simulink model "waypoint_generation_ptCloud_200726_mapdata_filtering_4m_2"  (R2020a)
settings: Solver=ode4  StartTime=0.0  StopTime=150  FixedStep=0.01  RelTol=1e-3  EnableMultiTasking=on
InitFcn:
  | detector = load('ptOPDetector.mat');
  | OPdetector = detector.OPdetector;
undefined symbols (not defined in the file): g, Kd_p, Kd_q, Kd_r, Kd_vx, Kd_vy, Kd_vz, Kff_r, Kff_vx, Kff_vy, Kff_vz, Ki_p, Ki_q, Ki_r, Ki_vx, Ki_vy, Ki_vz, Kp_p, Kp_phi, Kp_psi, Kp_q, Kp_r, Kp_theta, Kp_vx, Kp_vy, Kp_vz, M, pointCloud_center, sigma_motor, w_h
libraries: visiontextngfix x4, sharedtransform x1, shared6dof x1, simulink_extras x1
(part 1 of 3)
settings Model: Creator=WIN7  LastModifiedBy=USER
settings DataIOCC: LimitDataPoints=on  ReturnWorkspaceOutputs=off
settings OptimizationCC: LifeSpan=inf
settings DebuggingCC: AllowSymbolicDim=off  SFUnexpectedBacktrackingDiag=warning  SFNoUnconditionalDefaultTransitionDiag=warning  SFExecutionAtInitializationDiag=none  ArithmeticOperatorsInVariantConditions=warning
settings ModelReferenceCC: PropagateSignalLabelsOutOfModel=off
settings SFSimCC: SimUseLocalCustomCode=off  CustomCodeUndefinedFunction=UseInterfaceOnly
settings RTWCC: RTWUseLocalCustomCode=off
settings CodeAppCC: StateflowObjectComments=on
settings GRTTargetCC: TargetLangStandard=C89/C90 (ANSI)
settings ConfigComp: CovMetricSettings=dw  CovHtmlReporting=on  CovSaveCumulativeToWorkspaceVar=on  CovSaveSingleToWorkspaceVar=on  CovExternalEMLEnable=off

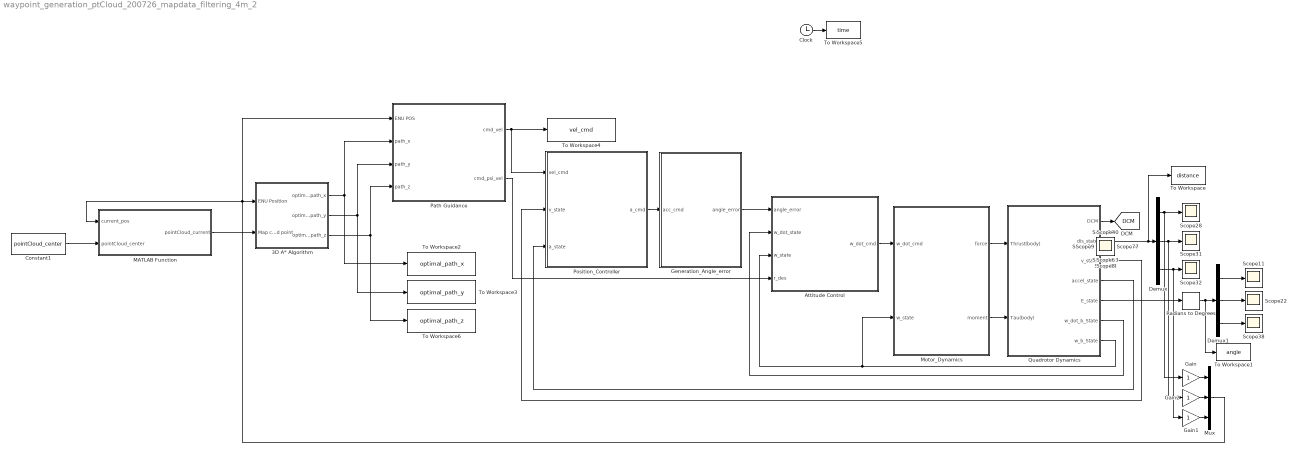
== system waypoint_generation_ptCloud_200726_mapdata_filtering_4m_2 ==
  3D A* Algorithm : Subsystem
  Attitude Control : Subsystem
  Clock : Clock
  Constant1 : Constant  Value=pointCloud_center
  Demux : Demux  Outputs=3
  Demux1 : Demux  Outputs=3
  Gain : Gain
  Gain1 : Gain
  Gain2 : Gain
  Generation_Angle_error : Subsystem
  MATLAB Function : MATLAB Function  TreatAsAtomicUnit=on
  Motor_Dynamics : Subsystem
  Mux : Mux  Inputs=3
  Path Guidance : Subsystem
  Position_Controller : Subsystem
  Quadrotor Dynamics : Subsystem
  Radians to Degrees : simulink_extras/Transformations/Radians to Degrees
  Scope{,1..40} (41 alike) : Scope
  To Workspace : ToWorkspace  VariableName=distance  SampleTime=-1
  To Workspace1 : ToWorkspace  VariableName=angle  SampleTime=-1
  To Workspace2 : ToWorkspace  VariableName=optimal_path_x  SampleTime=-1
  To Workspace3 : ToWorkspace  VariableName=optimal_path_y  SampleTime=-1
  To Workspace4 : ToWorkspace  VariableName=vel_cmd  SampleTime=-1
  To Workspace5 : ToWorkspace  VariableName=time  SampleTime=-1
  To Workspace6 : ToWorkspace  VariableName=optimal_path_z  SampleTime=-1
  tag scope: DCM=global
  wires:
  Quadrotor Dynamics/7(w_b_State) -> Attitude Control/3(w_state), Motor_Dynamics/2(w_state)
  Quadrotor Dynamics/6(w_dot_b_State) -> Attitude Control/2(w_dot_state)
  Quadrotor Dynamics/1(DCM) -> [DCM]
  Demux/1 -> Scope28/1, Gain/1
  Demux/3 -> Scope32/1, Gain1/1
  Demux/2 -> Scope31/1, Gain2/1
  Generation_Angle_error/1(angle_error) -> Attitude Control/1(angle_error)
  Position_Controller/1(a_cmd) -> Generation_Angle_error/1(acc_cmd)
  Quadrotor Dynamics/3(v_state) -> Position_Controller/2(v_state)
  Quadrotor Dynamics/4(accel_state) -> Position_Controller/3(a_state)
  Attitude Control/1(w_dot_cmd) -> Motor_Dynamics/1(w_dot_cmd)
  Motor_Dynamics/1(force) -> Quadrotor Dynamics/1(Thrust(body))
  Motor_Dynamics/2(moment) -> Quadrotor Dynamics/2(Tau(body))
  Demux1/1 -> Scope11/1
  Demux1/3 -> Scope38/1
  Demux1/2 -> Scope22/1
  Quadrotor Dynamics/5(E_state) -> Radians to Degrees/1
  Clock/1 -> To Workspace5/1
  Radians to Degrees/1 -> To Workspace1/1, Demux1/1
  Quadrotor Dynamics/2(dis_state) -> To Workspace/1, Demux/1
  Path Guidance/1(cmd_vel) -> Position_Controller/1("vel_cmd "), To Workspace4/1
  3D A* Algorithm/1(optimal_path_x) -> Path Guidance/2(path_x), To Workspace2/1
  3D A* Algorithm/2(optimal_path_y) -> Path Guidance/3(path_y), To Workspace3/1
  3D A* Algorithm/3(optimal_path_z) -> Path Guidance/4(path_z), To Workspace6/1
  Gain2/1 -> Mux/2
  Gain1/1 -> Mux/3
  Mux/1 -> Path Guidance/1("ENU POS "), MATLAB Function/1(current_pos), 3D A* Algorithm/1(ENU Position)
  Path Guidance/2("cmd_psi_vel ") -> Attitude Control/4("r_des ")
  Gain/1 -> Mux/1
  Constant1/1 -> MATLAB Function/2(pointCloud_center)
  MATLAB Function/1(pointCloud_current) -> 3D A* Algorithm/2(Map cloud point)

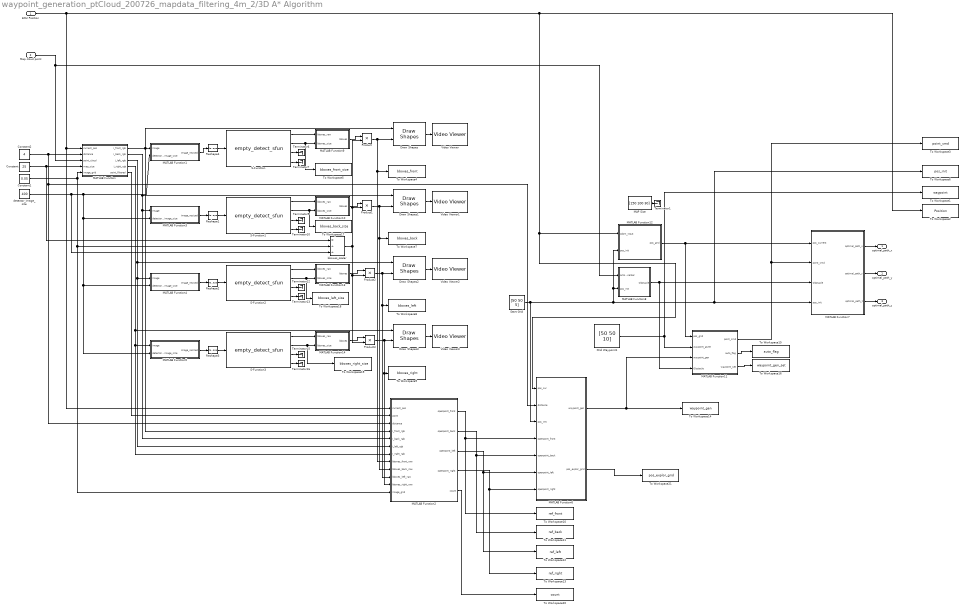
== system waypoint_generation_ptCloud_200726_mapdata_filtering_4m_2/3D A* Algorithm ==
  ENU Position : Inport
  Map cloud point : Inport  Port=2
  Constant : Constant  Value=25
  Constant1 : Constant  Value=0.05
  Constant2 : Constant  Value=4
  Draw Shapes{,1..3} (4 alike) : visiontextngfix/Draw Shapes  shape=Rectangles  fill=off  lineWidth=4  fillClrSource=Specify via dialog  display=User-specified value  intensity=200  color=[255 255 0]  opacity=0.6  viewport=Entire image  antialiasing=off  inType=Obsolete  imagePorts=One multidimensional signal  roundingMode=Floor  overflowMode=off  memoryMode=Specify word length  memoryWordLength=16  prodOutputMode=Binary point scaling  prodOutputWordLength=32  prodOutputFracLength=14  memoryFracLength=14
  Grid Waypoint1 : Constant  Value=[50 50 10]  VectorParams1D=off
  MAP Size : Constant  Value=[150 100 30]
  MATLAB Function : MATLAB Function  TreatAsAtomicUnit=on
  MATLAB Function1 : MATLAB Function  TreatAsAtomicUnit=on
  MATLAB Function10 : MATLAB Function  TreatAsAtomicUnit=on
  MATLAB Function11 : MATLAB Function  TreatAsAtomicUnit=on
  MATLAB Function12 : MATLAB Function  TreatAsAtomicUnit=on
  MATLAB Function13 : MATLAB Function  TreatAsAtomicUnit=on
  MATLAB Function14 : MATLAB Function  TreatAsAtomicUnit=on
  MATLAB Function2 : MATLAB Function  TreatAsAtomicUnit=on
  MATLAB Function3 : MATLAB Function  TreatAsAtomicUnit=on
  MATLAB Function4 : MATLAB Function  TreatAsAtomicUnit=on
  MATLAB Function5 : MATLAB Function  TreatAsAtomicUnit=on
  MATLAB Function6 : MATLAB Function  TreatAsAtomicUnit=on
  MATLAB Function7 : MATLAB Function  TreatAsAtomicUnit=on
  MATLAB Function8 : MATLAB Function  TreatAsAtomicUnit=on
  MATLAB Function9 : MATLAB Function  TreatAsAtomicUnit=on
  Product{,1..3} (4 alike) : Product
  Reshape{1..4} (4 alike) : Reshape
  S-Function{,1..3} (4 alike) : S-Function  FunctionName=empty_detect_sfun  SFunctionDeploymentMode=off  EnableBusSupport=off
  Start Grid : Constant  Value=[50 50 5]
  Terminator{1,6..7,9..10,12..13,15..16} (9 alike) : Terminator
  To Workspace1 : ToWorkspace  VariableName=waypoint  SampleTime=-1
      settings: Save2DSignal=2-D array (concatenate along first dimension)
  To Workspace10 : ToWorkspace  VariableName=ref_front  SampleTime=-1
  To Workspace11 : ToWorkspace  VariableName=ref_back  SampleTime=-1
  To Workspace12 : ToWorkspace  VariableName=ref_left  SampleTime=-1
  To Workspace13 : ToWorkspace  VariableName=ref_right  SampleTime=-1
  To Workspace14 : ToWorkspace  VariableName=waypoint_gen  SampleTime=-1
  To Workspace15 : ToWorkspace  VariableName=auto_flag  SampleTime=-1
  To Workspace16 : ToWorkspace  VariableName=waypoint_gen_set  SampleTime=-1
  To Workspace17 : ToWorkspace  VariableName=bboxes_back_size  SampleTime=-1
  To Workspace18 : ToWorkspace  VariableName=bboxes_left_size  SampleTime=-1
  To Workspace19 : ToWorkspace  VariableName=bboxes_right_size  SampleTime=-1
  To Workspace2 : ToWorkspace  VariableName=Position  SampleTime=-1
  To Workspace20 : ToWorkspace  VariableName=count  SampleTime=-1
  To Workspace21 : ToWorkspace  VariableName=pos_explor_grid  SampleTime=-1
  To Workspace3 : ToWorkspace  VariableName=point_cmd  SampleTime=-1
      settings: Save2DSignal=2-D array (concatenate along first dimension)
  To Workspace4 : ToWorkspace  VariableName=bboxes_front  SampleTime=-1
  To Workspace5 : ToWorkspace  VariableName=bboxes_front_size  SampleTime=-1
  To Workspace6 : ToWorkspace  VariableName=pos_init  SampleTime=-1
      settings: Save2DSignal=2-D array (concatenate along first dimension)
  To Workspace7 : ToWorkspace  VariableName=bboxes_back  SampleTime=-1
  To Workspace8 : ToWorkspace  VariableName=bboxes_left  SampleTime=-1
  To Workspace9 : ToWorkspace  VariableName=bboxes_right  SampleTime=-1
  Video Viewer : VideoViewer  FigPos=[7 678 732 569]
  Video Viewer1 : VideoViewer  FigPos=[742 680 732 569]
  Video Viewer2 : VideoViewer  FigPos=[0 1098 732 569]
  Video Viewer3 : VideoViewer  FigPos=[646 1041 732 569]
  bboxes_scalar : Product  Inputs=*//
  detector_image_size : Constant  Value=400
  optimal_path_x : Outport  VectorParamsAs1DForOutWhenUnconnected=off
  optimal_path_y : Outport  Port=2  VectorParamsAs1DForOutWhenUnconnected=off
  optimal_path_z : Outport  Port=3  VectorParamsAs1DForOutWhenUnconnected=off
  wires:
  MATLAB Function8/1(Obstacle) -> MATLAB Function11/4(Obstacle), MATLAB Function7/3(Obstacle)
  MATLAB Function12/1(pos_grid) -> MATLAB Function7/1(pos_current), MATLAB Function11/1(pos_grid)
  Start Grid/1 -> To Workspace6/1, MATLAB Function7/4(pos_init), MATLAB Function12/2(pos_init), MATLAB Function8/2(pos_init), MATLAB Function6/3(pos_init)
  MATLAB Function11/1(point_cmd) -> MATLAB Function7/2(point_cmd), To Workspace3/1
  MAP Size/1 -> Terminator1/1
  MATLAB Function7/1(optimal_path_x) -> optimal_path_x/1
  MATLAB Function7/2(optimal_path_y) -> optimal_path_y/1
  MATLAB Function7/3(optimal_path_z) -> optimal_path_z/1
  ENU Position/1 -> To Workspace2/1, MATLAB Function6/1(pos_cur), MATLAB Function12/1(odom_input), MATLAB Function2/1(current_pos), MATLAB Function/1(current_pos)
  Map cloud point/1 -> MATLAB Function8/1(octomap_center), MATLAB Function/3(point_cloud)
  Grid Waypoint1/1 -> To Workspace1/1, MATLAB Function11/2(waypoint_given)
  MATLAB Function/2(I_back_rgb) -> MATLAB Function2/5(I_back_rgb), MATLAB Function3/1(Image), Draw Shapes1/1
  MATLAB Function/3(I_left_rgb) -> MATLAB Function2/6(I_left_rgb), MATLAB Function4/1(Image), Draw Shapes2/1
  MATLAB Function1/1(Image_resized) -> Reshape4/1
  S-Function/2 -> To Workspace5/1, MATLAB Function9/2(bboxes_size)
  S-Function/4 -> Terminator7/1
  S-Function/3 -> Terminator6/1
  Reshape4/1 -> S-Function/1
  S-Function/1 -> MATLAB Function9/1(bboxes_raw)
  MATLAB Function/4(I_right_rgb) -> MATLAB Function2/7(I_right_rgb), MATLAB Function5/1(Image), Draw Shapes3/1
  S-Function1/3 -> Terminator9/1
  S-Function1/2 -> To Workspace17/1, MATLAB Function10/2(bboxes_size)
  MATLAB Function3/1(Image_resized) -> Reshape1/1
  S-Function1/4 -> Terminator10/1
  Reshape1/1 -> S-Function1/1
  S-Function1/1 -> MATLAB Function10/1(bboxes_raw)
  S-Function2/3 -> Terminator12/1
  S-Function2/2 -> To Workspace18/1, MATLAB Function13/2(bboxes_size)
  MATLAB Function4/1(Image_resized) -> Reshape2/1
  S-Function2/4 -> Terminator13/1
  Reshape2/1 -> S-Function2/1
  S-Function2/1 -> MATLAB Function13/1(bboxes_raw)
  S-Function3/3 -> Terminator15/1
  MATLAB Function5/1(Image_resized) -> Reshape3/1
  S-Function3/4 -> Terminator16/1
  Reshape3/1 -> S-Function3/1
  MATLAB Function2/4(openpoint_right) -> MATLAB Function6/7(openpoint_right), To Workspace13/1
  MATLAB Function2/3(openpoint_left) -> MATLAB Function6/6(openpoint_left), To Workspace12/1
  MATLAB Function2/1(openpoint_front) -> MATLAB Function6/4(openpoint_front), To Workspace10/1
  MATLAB Function2/2(openpoint_back) -> MATLAB Function6/5(openpoint_back), To Workspace11/1
  Draw Shapes/1 -> Video Viewer/1
  MATLAB Function/1(I_front_rgb) -> MATLAB Function2/4(I_front_rgb), Draw Shapes/1, MATLAB Function1/1(Image)
  Product/1 -> Draw Shapes/2, MATLAB Function2/8(bboxes_front_raw), To Workspace4/1
  Product1/1 -> MATLAB Function2/9(bboxes_back_raw), To Workspace7/1, Draw Shapes1/2
  Draw Shapes1/1 -> Video Viewer1/1
  Product2/1 -> Draw Shapes2/2, MATLAB Function2/10(bboxes_left_raw), To Workspace8/1
  Draw Shapes2/1 -> Video Viewer2/1
  Product3/1 -> Draw Shapes3/2, MATLAB Function2/11(bboxes_right_raw), To Workspace9/1
  Draw Shapes3/1 -> Video Viewer3/1
  MATLAB Function6/1(waypoint_gen) -> MATLAB Function11/3(waypoint_gen), To Workspace14/1
  MATLAB Function11/2(auto_flag) -> To Workspace15/1
  MATLAB Function11/3(waypoint_set) -> To Workspace16/1
  S-Function3/2 -> To Workspace19/1, MATLAB Function14/2(bboxes_size)
  S-Function3/1 -> MATLAB Function14/1(bboxes_raw)
  Constant/1 -> bboxes_scalar/1, MATLAB Function/4(map_size)
  Constant1/1 -> MATLAB Function2/12(image_grid), bboxes_scalar/2, MATLAB Function/5(image_grid)
  detector_image_size/1 -> bboxes_scalar/3, MATLAB Function5/2(detector_image_size), MATLAB Function4/2(detector_image_size), MATLAB Function3/2(detector_image_size), MATLAB Function1/2(detector_image_size)
  MATLAB Function9/1(bboxes) -> Product/1
  bboxes_scalar/1 -> Product3/2, Product2/2, Product1/2, Product/2
  MATLAB Function10/1(bboxes) -> Product1/1
  MATLAB Function13/1(bboxes) -> Product2/1
  MATLAB Function14/1(bboxes) -> Product3/1
  MATLAB Function2/5(count) -> To Workspace20/1
  MATLAB Function6/2(pos_explor_grid) -> To Workspace21/1
  Constant2/1 -> MATLAB Function6/2(distance), MATLAB Function2/3(distance), MATLAB Function/2(distance)
  MATLAB Function/5(point_filtered) -> MATLAB Function2/2(point)

== system waypoint_generation_ptCloud_200726_mapdata_filtering_4m_2/Attitude Control ==
  angle_error : Inport
  w_dot_state : Inport  Port=2
  w_state : Inport  Port=3
  "r_des " : Inport  Port=4
  Angle controller : Subsystem
  Angular velocity controller : Subsystem
  Mux1 : Mux  Inputs=3
  Step3 : Step  Time=0  After=0  SampleTime=0
  Step4 : Step  Time=0  After=0.002  SampleTime=0
  Step5 : Step  Time=0  After=0.005  SampleTime=0
  w_dot_cmd : Outport  VectorParamsAs1DForOutWhenUnconnected=off
  wires:
  angle_error/1 -> Angle controller/1(E_des)
  w_dot_state/1 -> Angular velocity controller/3(w_dot_state)
  w_state/1 -> Angular velocity controller/2(w_state)
  Step3/1 -> Mux1/1
  Step4/1 -> Mux1/2
  Step5/1 -> Mux1/3
  Angular velocity controller/1(w_dot_cmd) -> w_dot_cmd/1
  Angle controller/1(w_cmd) -> Angular velocity controller/1(w_cmd)
  "r_des "/1 -> Angular velocity controller/4("r_des ")

== system waypoint_generation_ptCloud_200726_mapdata_filtering_4m_2/Generation_Angle_error ==
  acc_cmd : Inport
  Attitude Generation (phi,theta,psi) : MATLAB Function  TreatAsAtomicUnit=on
  Attitude Generation(phi,theta,psi^*) : MATLAB Function  TreatAsAtomicUnit=on
  Attitude Generation(psi^*) : MATLAB Function  TreatAsAtomicUnit=on
  Constant : Constant  Value=0
  angle_error : Outport  VectorParamsAs1DForOutWhenUnconnected=off
  wires:
  [DCM] -> Attitude Generation (phi,theta,psi)/1(DCM)
  Attitude Generation (phi,theta,psi)/2(R_rp_x) -> Attitude Generation(psi^*)/1(R_rp_x)
  acc_cmd/1 -> Attitude Generation(psi^*)/2(acc_cmd), Attitude Generation (phi,theta,psi)/2(acc_cmd)
  Attitude Generation(phi,theta,psi^*)/1(angle_error_result) -> angle_error/1
  Attitude Generation (phi,theta,psi)/1(angle_error) -> Attitude Generation(phi,theta,psi^*)/1(angle_error)
  Attitude Generation(psi^*)/1(psi_angle_error) -> Attitude Generation(phi,theta,psi^*)/2(psi_angle_error)
  Constant/1 -> Attitude Generation(psi^*)/3(Bearing_angle)

== system waypoint_generation_ptCloud_200726_mapdata_filtering_4m_2/Motor_Dynamics ==
  w_dot_cmd : Inport
  w_state : Inport  Port=2
  Motor Dynamics : Subsystem
  "Thrust &  Moment Generation " : MATLAB Function  TreatAsAtomicUnit=on
  force : Outport  VectorParamsAs1DForOutWhenUnconnected=off
  moment : Outport  Port=2  VectorParamsAs1DForOutWhenUnconnected=off
  wires:
  "Thrust &  Moment Generation "/2(moment) -> moment/1
  "Thrust &  Moment Generation "/1(force) -> force/1
  Motor Dynamics/1(w_com) -> "Thrust &  Moment Generation "/1(w_des_nomal)
  w_dot_cmd/1 -> Motor Dynamics/1(w_dot_cmd)
  w_state/1 -> Motor Dynamics/2(w_state)

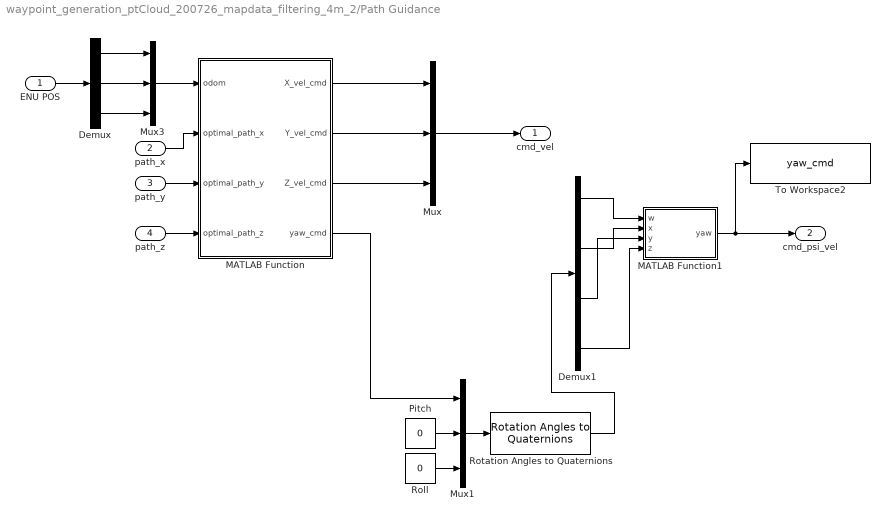
== system waypoint_generation_ptCloud_200726_mapdata_filtering_4m_2/Path Guidance ==
  "ENU POS " : Inport
  path_x : Inport  Port=2
  path_y : Inport  Port=3
  path_z : Inport  Port=4
  " Roll" : Constant  Value=0  OutDataTypeStr=double  SampleTime=-1
  Demux : Demux  Outputs=3
  Demux1 : Demux
  MATLAB Function : MATLAB Function  TreatAsAtomicUnit=on
  MATLAB Function1 : MATLAB Function  TreatAsAtomicUnit=on
  Mux : Mux  Inputs=3
  Mux1 : Mux  Inputs=3
  Mux3 : Mux  Inputs=3
  Pitch : Constant  Value=0  OutDataTypeStr=double  SampleTime=-1
  Rotation Angles to Quaternions : sharedtransform/Rotation Angles to Quaternions  rotationOrder=ZYX  aMode=aMode
      settings: SourceProductBaseCode=AE,PW,MT,VE,VP
  To Workspace2 : ToWorkspace  VariableName=yaw_cmd  SampleTime=-1
  cmd_vel : Outport  VectorParamsAs1DForOutWhenUnconnected=off
  "cmd_psi_vel " : Outport  Port=2  VectorParamsAs1DForOutWhenUnconnected=off
  wires:
  MATLAB Function/3(Z_vel_cmd) -> Mux/3
  path_y/1 -> MATLAB Function/3(optimal_path_y)
  Mux3/1 -> MATLAB Function/1(odom)
  path_z/1 -> MATLAB Function/4(optimal_path_z)
  path_x/1 -> MATLAB Function/2(optimal_path_x)
  Mux/1 -> cmd_vel/1
  "ENU POS "/1 -> Demux/1
  Demux/1 -> Mux3/1
  Demux/2 -> Mux3/2
  Demux/3 -> Mux3/3
  MATLAB Function/1(X_vel_cmd) -> Mux/1
  MATLAB Function/2(Y_vel_cmd) -> Mux/2
  Demux1/4 -> MATLAB Function1/4(z)
  " Roll"/1 -> Mux1/3
  Mux1/1 -> Rotation Angles to Quaternions/1
  MATLAB Function/4(yaw_cmd) -> Mux1/1
  Pitch/1 -> Mux1/2
  Rotation Angles to Quaternions/1 -> Demux1/1
  Demux1/3 -> MATLAB Function1/3(y)
  Demux1/1 -> MATLAB Function1/1(w)
  Demux1/2 -> MATLAB Function1/2(x)
  MATLAB Function1/1(yaw) -> To Workspace2/1, "cmd_psi_vel "/1

== system waypoint_generation_ptCloud_200726_mapdata_filtering_4m_2/Position_Controller ==
  "vel_cmd " : Inport
  v_state : Inport  Port=2
  a_state : Inport  Port=3
  Velocity Controller : Subsystem
  a_cmd : Outport  VectorParamsAs1DForOutWhenUnconnected=off
  wires:
  Velocity Controller/1(a_cmd) -> a_cmd/1
  v_state/1 -> Velocity Controller/2(v_state)
  a_state/1 -> Velocity Controller/3(a_state)
  "vel_cmd "/1 -> Velocity Controller/1(v_cmd)

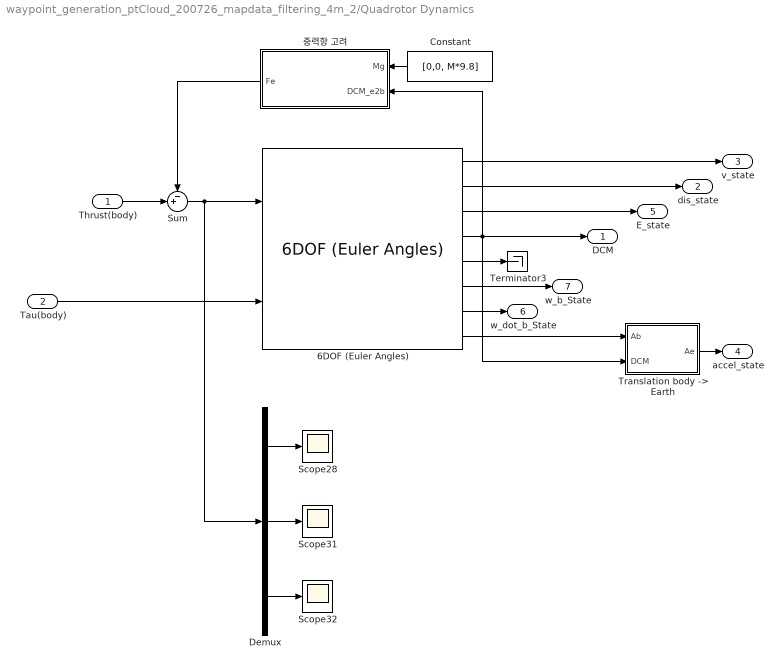
== system waypoint_generation_ptCloud_200726_mapdata_filtering_4m_2/Quadrotor Dynamics ==
  Thrust(body) : Inport
  Tau(body) : Inport  Port=2
  6DOF (Euler Angles) : shared6dof/6DOF (Euler Angles)  units=Metric (MKS)  mtype=Fixed  rep=Euler Angles  xme_0=initial_position  Vm_0=initial_velocity  eul_0=[0 0 0]  pm_0=[0 0 0]  mass_0=M  mass_e=0.5  mass_f=2.0  inertia=Inertia  inertia_e=eye(3)  inertia_f=2*eye(3)  k_quat=1.0  vre_flag=on  abi_flag=off  aMode=aMode  xme_statename=''  Vm_statename=''  eul_statename=''  quat_statename=''  pm_statename=''  mass_statename=''
      settings: SourceProductBaseCode=AE,PW,MT,VE,VP
  Constant : Constant  Value=[0,0, M*9.8]
  Demux : Demux  Outputs=3
  Scope28 : Scope
  Scope31 : Scope
  Scope32 : Scope
  Sum : Sum  Inputs=-+|
  Terminator3 : Terminator
  "Translation body -> Earth" : MATLAB Function  TreatAsAtomicUnit=on
  중력항 고려 : MATLAB Function  TreatAsAtomicUnit=on
  DCM : Outport  VectorParamsAs1DForOutWhenUnconnected=off
  dis_state : Outport  Port=2  VectorParamsAs1DForOutWhenUnconnected=off
  v_state : Outport  Port=3  VectorParamsAs1DForOutWhenUnconnected=off
  accel_state : Outport  Port=4  VectorParamsAs1DForOutWhenUnconnected=off
  E_state : Outport  Port=5  VectorParamsAs1DForOutWhenUnconnected=off
  w_dot_b_State : Outport  Port=6  VectorParamsAs1DForOutWhenUnconnected=off
  w_b_State : Outport  Port=7  VectorParamsAs1DForOutWhenUnconnected=off
  wires:
  Constant/1 -> 중력항 고려/1(Mg)
  6DOF (Euler Angles)/4 -> 중력항 고려/2(DCM_e2b), DCM/1, "Translation body -> Earth"/2(DCM)
  Thrust(body)/1 -> Sum/2
  6DOF (Euler Angles)/5 -> Terminator3/1
  6DOF (Euler Angles)/1 -> v_state/1
  6DOF (Euler Angles)/7 -> w_dot_b_State/1
  중력항 고려/1(Fe) -> Sum/1
  Tau(body)/1 -> 6DOF (Euler Angles)/2
  6DOF (Euler Angles)/6 -> w_b_State/1
  "Translation body -> Earth"/1(Ae) -> accel_state/1
  6DOF (Euler Angles)/8 -> "Translation body -> Earth"/1(Ab)
  6DOF (Euler Angles)/3 -> E_state/1
  6DOF (Euler Angles)/2 -> dis_state/1
  Sum/1 -> Demux/1, 6DOF (Euler Angles)/1
  Demux/1 -> Scope28/1
  Demux/3 -> Scope32/1
  Demux/2 -> Scope31/1

== system waypoint_generation_ptCloud_200726_mapdata_filtering_4m_2/Attitude Control/Angle controller ==
  E_des : Inport
  Mux : Mux  Inputs=3
  p_controller : Subsystem
  p_controller1 : Subsystem
  p_controller2 : Subsystem
  w_cmd : Outport  VectorParamsAs1DForOutWhenUnconnected=off
  wires:
  E_des/1 -> p_controller2/1(psi_des), p_controller1/1(theta_des), p_controller/1(phi_des)
  p_controller1/1(q_des) -> Mux/2
  p_controller/1(p_des) -> Mux/1
  p_controller2/1(r_des) -> Mux/3
  Mux/1 -> w_cmd/1

== system waypoint_generation_ptCloud_200726_mapdata_filtering_4m_2/Attitude Control/Angular velocity controller ==
  note: desired angular accelation
  w_cmd : Inport
  w_state : Inport  Port=2
  w_dot_state : Inport  Port=3
  "r_des " : Inport  Port=4
  Constant2 : Constant  Value=0
  Constant3 : Constant  Value=0
  Constant4 : Constant  Value=0
  Gain : Gain  Gain=50
  Gain1 : Gain  Gain=50
  Mux : Mux  Inputs=3
  Mux1 : Mux  Inputs=3
  p_dot_controller : Subsystem
  q_dot_controller : Subsystem
  r_dot_controller : Subsystem
  w_dot_cmd : Outport  VectorParamsAs1DForOutWhenUnconnected=off
  wires:
  p_dot_controller/1(p_dot) -> Gain/1
  q_dot_controller/1(q_dot) -> Gain1/1
  w_state/1 -> r_dot_controller/2(r_state), q_dot_controller/2(q_state), p_dot_controller/2(p_state)
  w_dot_state/1 -> p_dot_controller/4(p_dot_state), q_dot_controller/4(q_dot_state), r_dot_controller/4(r_dot_state)
  Constant2/1 -> Mux1/1
  Constant3/1 -> Mux1/2
  Constant4/1 -> Mux1/3
  w_cmd/1 -> q_dot_controller/1(q_des), p_dot_controller/1(p_des)
  Mux/1 -> w_dot_cmd/1
  Mux1/1 -> r_dot_controller/3(r_dot_des), q_dot_controller/3(q_dot_des), p_dot_controller/3(p_dot_des)
  Gain/1 -> Mux/1
  Gain1/1 -> Mux/2
  r_dot_controller/1(r_dot) -> Mux/3
  "r_des "/1 -> r_dot_controller/1(r_des)

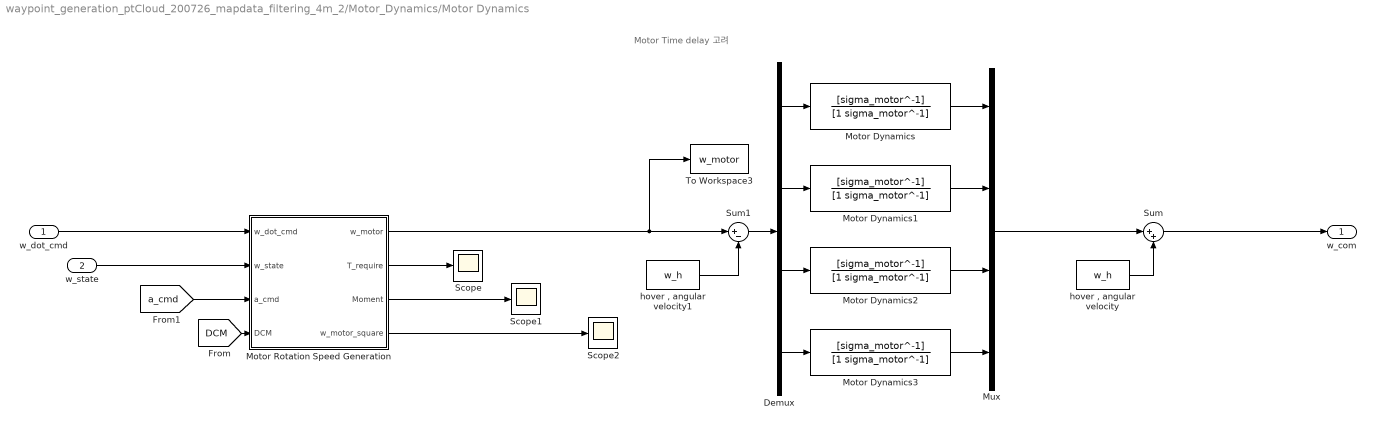
== system waypoint_generation_ptCloud_200726_mapdata_filtering_4m_2/Motor_Dynamics/Motor Dynamics ==
  note: Motor Time delay 고려
  w_dot_cmd : Inport
  w_state : Inport  Port=2
  Demux : Demux
  Motor Dynamics{,1..3} (4 alike) : TransferFcn  Numerator=[sigma_motor^-1]  Denominator=[1 sigma_motor^-1]
  Motor Rotation Speed Generation : MATLAB Function  TreatAsAtomicUnit=on
  Mux : Mux
  Scope : Scope
  Scope1 : Scope
  Scope2 : Scope
  Sum : Sum  Inputs=|++
  Sum1 : Sum  Inputs=|+-
  To Workspace3 : ToWorkspace  VariableName=w_motor  SampleTime=-1
  "hover , angular velocity" : Constant  Value=w_h
  "hover , angular velocity1" : Constant  Value=w_h
  w_com : Outport  VectorParamsAs1DForOutWhenUnconnected=off
  wires:
  Demux/2 -> Motor Dynamics1/1
  Demux/1 -> Motor Dynamics/1
  Demux/3 -> Motor Dynamics2/1
  Demux/4 -> Motor Dynamics3/1
  Motor Dynamics2/1 -> Mux/3
  Motor Dynamics3/1 -> Mux/4
  Motor Dynamics/1 -> Mux/1
  Motor Dynamics1/1 -> Mux/2
  Mux/1 -> Sum/1
  Sum/1 -> w_com/1
  "hover , angular velocity"/1 -> Sum/2
  Sum1/1 -> Demux/1
  "hover , angular velocity1"/1 -> Sum1/2
  Motor Rotation Speed Generation/1(w_motor) -> To Workspace3/1, Sum1/1
  w_dot_cmd/1 -> Motor Rotation Speed Generation/1(w_dot_cmd)
  w_state/1 -> Motor Rotation Speed Generation/2(w_state)
  Motor Rotation Speed Generation/2(T_require) -> Scope/1
  Motor Rotation Speed Generation/3(Moment) -> Scope1/1
  Motor Rotation Speed Generation/4(w_motor_square) -> Scope2/1
  [a_cmd] -> Motor Rotation Speed Generation/3(a_cmd)
  [DCM] -> Motor Rotation Speed Generation/4(DCM)

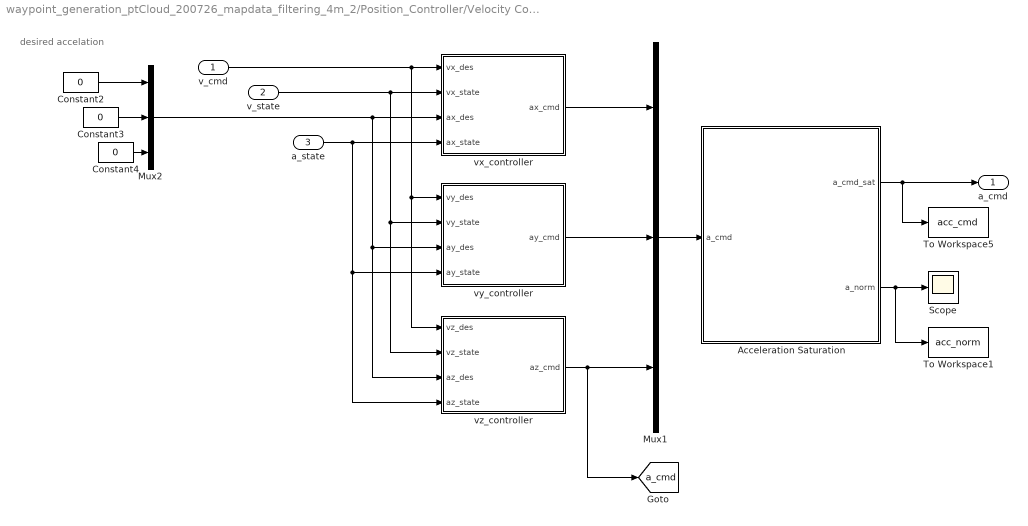
== system waypoint_generation_ptCloud_200726_mapdata_filtering_4m_2/Position_Controller/Velocity Controller ==
  note: desired accelation
  v_cmd : Inport
  v_state : Inport  Port=2
  a_state : Inport  Port=3
  Acceleration Saturation : MATLAB Function  TreatAsAtomicUnit=on
  Constant2 : Constant  Value=0
  Constant3 : Constant  Value=0
  Constant4 : Constant  Value=0
  Mux1 : Mux  Inputs=3
  Mux2 : Mux  Inputs=3
  Scope : Scope
  To Workspace1 : ToWorkspace  VariableName=acc_norm  SampleTime=-1
  To Workspace5 : ToWorkspace  VariableName=acc_cmd  SampleTime=-1
  vx_controller : Subsystem
  vy_controller : Subsystem
  vz_controller : Subsystem
  a_cmd : Outport  VectorParamsAs1DForOutWhenUnconnected=off
  tag scope: a_cmd=global
  wires:
  Constant2/1 -> Mux2/1
  Mux2/1 -> vx_controller/3(ax_des), vy_controller/3(ay_des), vz_controller/3(az_des)
  v_state/1 -> vx_controller/2(vx_state), vy_controller/2(vy_state), vz_controller/2(vz_state)
  Constant4/1 -> Mux2/3
  Constant3/1 -> Mux2/2
  v_cmd/1 -> vx_controller/1(vx_des), vy_controller/1(vy_des), vz_controller/1(vz_des)
  vx_controller/1(ax_cmd) -> Mux1/1
  vy_controller/1(ay_cmd) -> Mux1/2
  a_state/1 -> vy_controller/4(ay_state), vz_controller/4(az_state), vx_controller/4(ax_state)
  vz_controller/1(az_cmd) -> [a_cmd], Mux1/3
  Mux1/1 -> Acceleration Saturation/1(a_cmd)
  Acceleration Saturation/1(a_cmd_sat) -> To Workspace5/1, a_cmd/1
  Acceleration Saturation/2(a_norm) -> To Workspace1/1, Scope/1

== system waypoint_generation_ptCloud_200726_mapdata_filtering_4m_2/Attitude Control/Angle controller/p_controller ==
  phi_des : Inport
  Gain : Gain  Gain=Kp_phi
  Selector : Selector  InputPortWidth=3  IndexOptions=Index vector (dialog)  Indices=[1]  OutputSizes=1
  p_des : Outport  VectorParamsAs1DForOutWhenUnconnected=off
  wires:
  phi_des/1 -> Selector/1
  Selector/1 -> Gain/1
  Gain/1 -> p_des/1

== system waypoint_generation_ptCloud_200726_mapdata_filtering_4m_2/Attitude Control/Angle controller/p_controller1 ==
  theta_des : Inport
  Gain : Gain  Gain=Kp_theta
  Selector : Selector  InputPortWidth=3  IndexOptions=Index vector (dialog)  Indices=[2]  OutputSizes=1
  q_des : Outport  VectorParamsAs1DForOutWhenUnconnected=off
  wires:
  Selector/1 -> Gain/1
  theta_des/1 -> Selector/1
  Gain/1 -> q_des/1

== system waypoint_generation_ptCloud_200726_mapdata_filtering_4m_2/Attitude Control/Angle controller/p_controller2 ==
  psi_des : Inport
  Gain : Gain  Gain=Kp_psi
  Selector : Selector  InputPortWidth=3  IndexOptions=Index vector (dialog)  Indices=[3]  OutputSizes=1
  r_des : Outport  VectorParamsAs1DForOutWhenUnconnected=off
  wires:
  psi_des/1 -> Selector/1
  Gain/1 -> r_des/1
  Selector/1 -> Gain/1

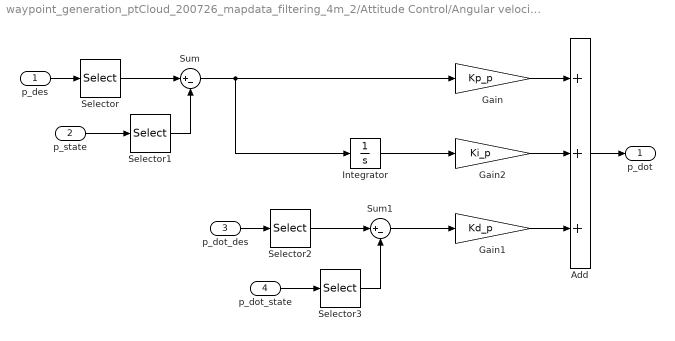
== system waypoint_generation_ptCloud_200726_mapdata_filtering_4m_2/Attitude Control/Angular velocity controller/p_dot_controller ==
  p_des : Inport
  p_state : Inport  Port=2
  p_dot_des : Inport  Port=3
  p_dot_state : Inport  Port=4
  Add : Sum  Inputs=+++
  Gain : Gain  Gain=Kp_p
  Gain1 : Gain  Gain=Kd_p
  Gain2 : Gain  Gain=Ki_p
  Integrator : Integrator
  Selector{,1..3} (4 alike) : Selector  InputPortWidth=3  IndexOptions=Index vector (dialog)  Indices=[1]  OutputSizes=1
  Sum : Sum  Inputs=|+-
  Sum1 : Sum  Inputs=|+-
  p_dot : Outport  VectorParamsAs1DForOutWhenUnconnected=off
  wires:
  p_des/1 -> Selector/1
  p_state/1 -> Selector1/1
  p_dot_des/1 -> Selector2/1
  p_dot_state/1 -> Selector3/1
  Sum/1 -> Gain/1, Integrator/1
  Sum1/1 -> Gain1/1
  Gain/1 -> Add/1
  Add/1 -> p_dot/1
  Selector/1 -> Sum/1
  Selector1/1 -> Sum/2
  Selector2/1 -> Sum1/1
  Selector3/1 -> Sum1/2
  Gain1/1 -> Add/3
  Integrator/1 -> Gain2/1
  Gain2/1 -> Add/2

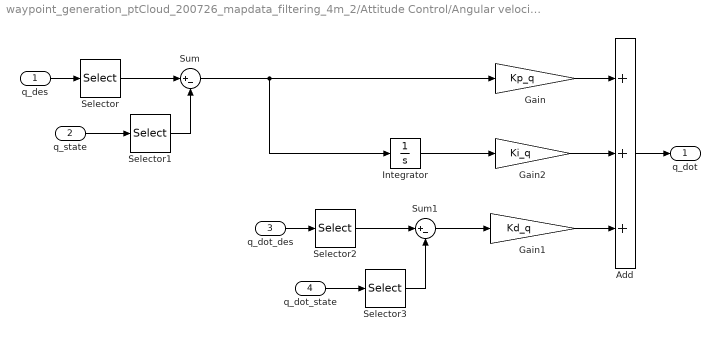
== system waypoint_generation_ptCloud_200726_mapdata_filtering_4m_2/Attitude Control/Angular velocity controller/q_dot_controller ==
  q_des : Inport
  q_state : Inport  Port=2
  q_dot_des : Inport  Port=3
  q_dot_state : Inport  Port=4
  Add : Sum  Inputs=+++
  Gain : Gain  Gain=Kp_q
  Gain1 : Gain  Gain=Kd_q
  Gain2 : Gain  Gain=Ki_q
  Integrator : Integrator
  Selector{,1..3} (4 alike) : Selector  InputPortWidth=3  IndexOptions=Index vector (dialog)  Indices=[2]  OutputSizes=1
  Sum : Sum  Inputs=|+-
  Sum1 : Sum  Inputs=|+-
  q_dot : Outport  VectorParamsAs1DForOutWhenUnconnected=off
  wires:
  q_des/1 -> Selector/1
  q_state/1 -> Selector1/1
  q_dot_des/1 -> Selector2/1
  q_dot_state/1 -> Selector3/1
  Sum/1 -> Integrator/1, Gain/1
  Sum1/1 -> Gain1/1
  Gain/1 -> Add/1
  Add/1 -> q_dot/1
  Selector/1 -> Sum/1
  Selector1/1 -> Sum/2
  Selector2/1 -> Sum1/1
  Selector3/1 -> Sum1/2
  Gain1/1 -> Add/3
  Gain2/1 -> Add/2
  Integrator/1 -> Gain2/1

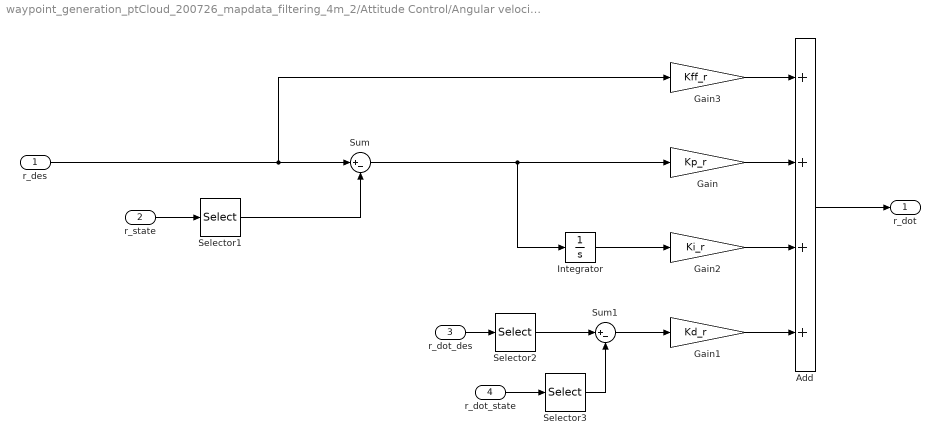
== system waypoint_generation_ptCloud_200726_mapdata_filtering_4m_2/Attitude Control/Angular velocity controller/r_dot_controller ==
  r_des : Inport
  r_state : Inport  Port=2
  r_dot_des : Inport  Port=3
  r_dot_state : Inport  Port=4
  Add : Sum  Inputs=++++
  Gain : Gain  Gain=Kp_r
  Gain1 : Gain  Gain=Kd_r
  Gain2 : Gain  Gain=Ki_r
  Gain3 : Gain  Gain=Kff_r
  Integrator : Integrator
  Selector1 : Selector  InputPortWidth=3  IndexOptions=Index vector (dialog)  Indices=[3]  OutputSizes=1
  Selector2 : Selector  InputPortWidth=3  IndexOptions=Index vector (dialog)  Indices=[3]  OutputSizes=1
  Selector3 : Selector  InputPortWidth=3  IndexOptions=Index vector (dialog)  Indices=[3]  OutputSizes=1
  Sum : Sum  Inputs=|+-
  Sum1 : Sum  Inputs=|+-
  r_dot : Outport  VectorParamsAs1DForOutWhenUnconnected=off
  wires:
  Selector3/1 -> Sum1/2
  Selector2/1 -> Sum1/1
  Selector1/1 -> Sum/2
  r_des/1 -> Gain3/1, Sum/1
  Add/1 -> r_dot/1
  Gain/1 -> Add/2
  Sum1/1 -> Gain1/1
  Sum/1 -> Integrator/1, Gain/1
  r_dot_state/1 -> Selector3/1
  r_dot_des/1 -> Selector2/1
  r_state/1 -> Selector1/1
  Gain1/1 -> Add/4
  Gain2/1 -> Add/3
  Integrator/1 -> Gain2/1
  Gain3/1 -> Add/1

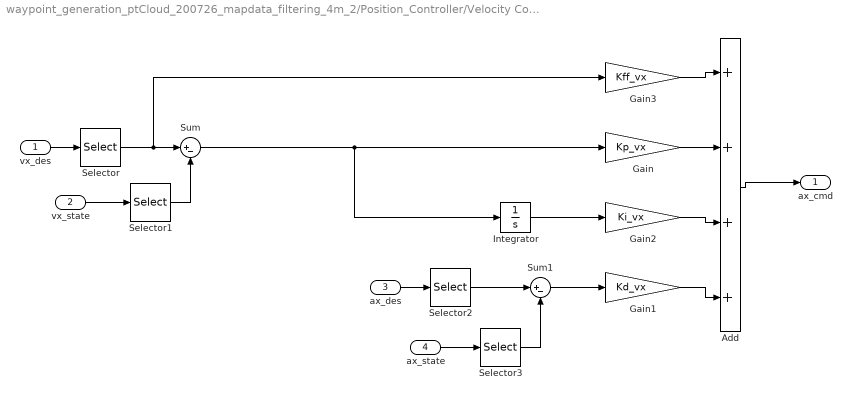
== system waypoint_generation_ptCloud_200726_mapdata_filtering_4m_2/Position_Controller/Velocity Controller/vx_controller ==
  vx_des : Inport
  vx_state : Inport  Port=2
  ax_des : Inport  Port=3
  ax_state : Inport  Port=4
  Add : Sum  Inputs=++++
  Gain : Gain  Gain=Kp_vx
  Gain1 : Gain  Gain=Kd_vx
  Gain2 : Gain  Gain=Ki_vx
  Gain3 : Gain  Gain=Kff_vx
  Integrator : Integrator
  Selector{,1..3} (4 alike) : Selector  InputPortWidth=3  IndexOptions=Index vector (dialog)  Indices=[1]  OutputSizes=1
  Sum : Sum  Inputs=|+-
  Sum1 : Sum  Inputs=|+-
  ax_cmd : Outport  VectorParamsAs1DForOutWhenUnconnected=off
  wires:
  vx_des/1 -> Selector/1
  vx_state/1 -> Selector1/1
  ax_des/1 -> Selector2/1
  ax_state/1 -> Selector3/1
  Sum/1 -> Integrator/1, Gain/1
  Sum1/1 -> Gain1/1
  Gain/1 -> Add/2
  Add/1 -> ax_cmd/1
  Selector/1 -> Gain3/1, Sum/1
  Selector1/1 -> Sum/2
  Selector2/1 -> Sum1/1
  Selector3/1 -> Sum1/2
  Gain1/1 -> Add/4
  Integrator/1 -> Gain2/1
  Gain2/1 -> Add/3
  Gain3/1 -> Add/1

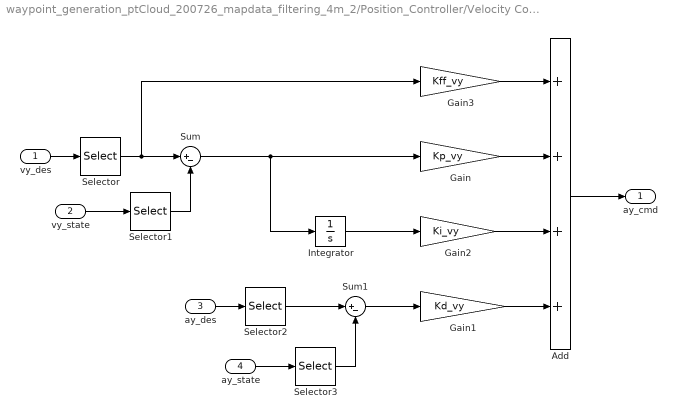
== system waypoint_generation_ptCloud_200726_mapdata_filtering_4m_2/Position_Controller/Velocity Controller/vy_controller ==
  vy_des : Inport
  vy_state : Inport  Port=2
  ay_des : Inport  Port=3
  ay_state : Inport  Port=4
  Add : Sum  Inputs=++++
  Gain : Gain  Gain=Kp_vy
  Gain1 : Gain  Gain=Kd_vy
  Gain2 : Gain  Gain=Ki_vy
  Gain3 : Gain  Gain=Kff_vy
  Integrator : Integrator
  Selector{,1..3} (4 alike) : Selector  InputPortWidth=3  IndexOptions=Index vector (dialog)  Indices=[2]  OutputSizes=1
  Sum : Sum  Inputs=|+-
  Sum1 : Sum  Inputs=|+-
  ay_cmd : Outport  VectorParamsAs1DForOutWhenUnconnected=off
  wires:
  Add/1 -> ay_cmd/1
  vy_des/1 -> Selector/1
  vy_state/1 -> Selector1/1
  ay_des/1 -> Selector2/1
  ay_state/1 -> Selector3/1
  Sum/1 -> Integrator/1, Gain/1
  Sum1/1 -> Gain1/1
  Selector/1 -> Gain3/1, Sum/1
  Selector1/1 -> Sum/2
  Selector2/1 -> Sum1/1
  Selector3/1 -> Sum1/2
  Integrator/1 -> Gain2/1
  Gain/1 -> Add/2
  Gain2/1 -> Add/3
  Gain1/1 -> Add/4
  Gain3/1 -> Add/1

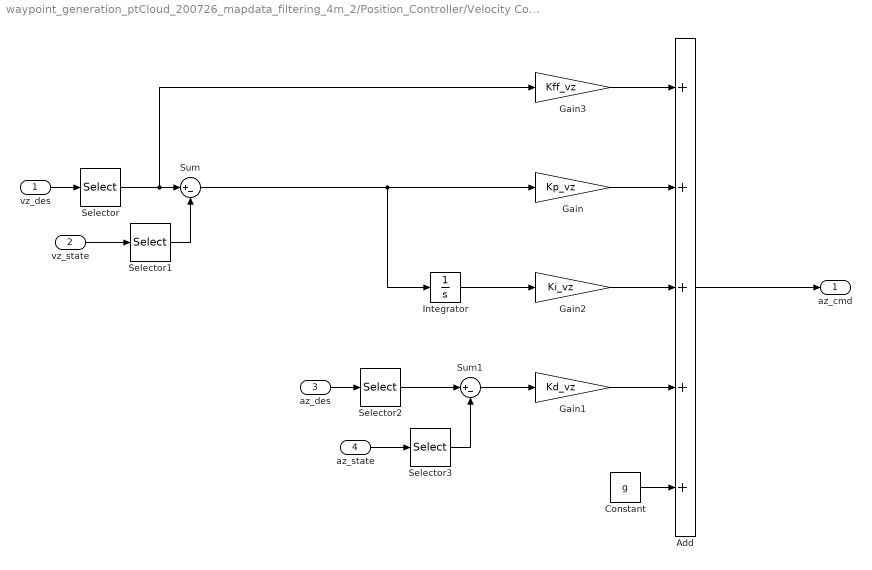
== system waypoint_generation_ptCloud_200726_mapdata_filtering_4m_2/Position_Controller/Velocity Controller/vz_controller ==
  vz_des : Inport
  vz_state : Inport  Port=2
  az_des : Inport  Port=3
  az_state : Inport  Port=4
  Add : Sum  Inputs=+++++
  Constant : Constant  Value=g
  Gain : Gain  Gain=Kp_vz
  Gain1 : Gain  Gain=Kd_vz
  Gain2 : Gain  Gain=Ki_vz
  Gain3 : Gain  Gain=Kff_vz
  Integrator : Integrator
  Selector{,1..3} (4 alike) : Selector  InputPortWidth=3  IndexOptions=Index vector (dialog)  Indices=[3]  OutputSizes=1
  Sum : Sum  Inputs=|+-
  Sum1 : Sum  Inputs=|+-
  az_cmd : Outport  VectorParamsAs1DForOutWhenUnconnected=off
  wires:
  Selector3/1 -> Sum1/2
  Selector2/1 -> Sum1/1
  Selector1/1 -> Sum/2
  Selector/1 -> Gain3/1, Sum/1
  Gain/1 -> Add/2
  az_state/1 -> Selector3/1
  az_des/1 -> Selector2/1
  vz_state/1 -> Selector1/1
  vz_des/1 -> Selector/1
  Sum/1 -> Integrator/1, Gain/1
  Sum1/1 -> Gain1/1
  Add/1 -> az_cmd/1
  Integrator/1 -> Gain2/1
  Gain2/1 -> Add/3
  Gain1/1 -> Add/4
  Constant/1 -> Add/5
  Gain3/1 -> Add/1

== matlab function waypoint_generation_ptCloud_200726_mapdata_filtering_4m_2/3D A* Algorithm/MATLAB Function ==
  settings: updateMethod=DISCRETE
  data: current_pos input; distance input; point_cloud input; I_front_rgb output; I_back_rgb output; I_left_rgb output; I_right_rgb output; map_size input; image_grid input; point_filtered output
function [I_front_rgb,I_back_rgb,I_left_rgb,I_right_rgb,point_filtered] = fcn(current_pos,distance,point_cloud,map_size,image_grid)

% persistent image_hz image_temp_front image_temp_back image_temp_left image_temp_right
% distance=6;
    pos_x = current_pos(1);
    pos_y = current_pos(2);
    pos_z = current_pos(3);
    
for lll=1:numel(point_cloud)/3
    if sqrt((point_cloud(lll,1)-pos_x)^2 + (point_cloud(lll,2)-pos_y)^2 + (point_cloud(lll,3)-pos_z)^2) > distance
        point_cloud(lll,:)=nan(1,3);
    else
        point_cloud(lll,:)=[point_cloud(lll,1)-pos_x, point_cloud(lll,2)-pos_y, point_cloud(lll,3)-pos_z];
    end
end

point = rmmissing(point_cloud);

% test_size = 25;                             % -12.5m ~ 12.5m
% map_size = 50;                             % -25m ~ 25m
% test_grid = 0.02;                         %m
% image_grid = 0.10;                           %m
% test_grid = 0.1;                          %m

image_size = map_size/image_grid;           %
image_size = 500;
% image_size = 1000;                        % 이미지 4개 만드는데 10초
% image_size = 400;                         % 이미지 4개 만드는데 1.6초
% image_size = 200;                         % 이미지 4개 만드는데 0.5초

% if isempty(image_hz)
%     image_hz = 299;
% end
% if isempty(image_temp_front)
%     image_temp_front = single(cat(3,zeros(image_size,image_size),zeros(image_size,image_size),zeros(image_size,image_size)));
% end
% if isempty(image_temp_back)
%     image_temp_back = single(cat(3,zeros(image_size,image_size),zeros(image_size,image_size),zeros(image_size,image_size)));
% end
% if isempty(image_temp_left)
%     image_temp_left = single(cat(3,zeros(image_size,image_size),zeros(image_size,image_size),zeros(image_size,image_size)));
% end
% if isempty(image_temp_right)
%     image_temp_right = single(cat(3,zeros(image_size,image_size),zeros(image_size,image_size),zeros(image_size,image_size)));
% end
% 
% image_hz = image_hz + 1;
% 
% % tic
% if image_hz == 300
%     image_hz = 1;


% indices_front = cell(image_size,image_size);
% indices_back = cell(image_size,image_size);
% indices_right = cell(image_size,image_size);
% indices_left = cell(image_size,image_size);
indices_front = zeros(image_size,image_size);
indices_back = zeros(image_size,image_size);
indices_right = zeros(image_size,image_size);
indices_left = zeros(image_size,image_size);

% if ~(current_pos(1) == 0 && current_pos(2) == 0 && current_pos(3) == 0)
    
    size = numel(point)/3;
    point_shifted = point+image_size*image_grid/2;
    % point_grided = int16(point.Location/test_grid);
    point_grided = int16(point_shifted/image_grid);
%     
%     current_x = pos_x/test_grid;
%     current_y = pos_y/test_grid;
%     current_z = pos_z/test_grid;
%     
%     for aa = 1:size
%         if point(aa,1) >= pos_x
%             indices_front{point_grided(aa,3),point_grided(aa,2)}=[indices_front{point_grided(aa,3),point_grided(aa,2)};aa];
%         elseif point(aa,1) <= pos_x
%             indices_back{point_grided(aa,3),point_grided(aa,2)}=[indices_back{point_grided(aa,3),point_grided(aa,2)};aa];
%         end
%         
%         if point(aa,2) >= pos_y
%             indices_left{point_grided(aa,3),point_grided(aa,1)}=[indices_left{point_grided(aa,3),point_grided(aa,1)};aa];
%         elseif point(aa,2) <= pos_y
%             indices_right{point_grided(aa,3),point_grided(aa,1)}=[indices_right{point_grided(aa,3),point_grided(aa,1)};aa];
%         end
%     end
    
    for aa = 1:size
%         if point(aa,1) >= pos_x
        if point(aa,1) >= 0
            indices_front(point_grided(aa,3),point_grided(aa,2))=1;
%         elseif point(aa,1) <= pos_x
        elseif point(aa,1) <= 0
            indices_back(point_grided(aa,3),point_grided(aa,2))=1;
        end
        
%         if point(aa,2) >= pos_y
        if point(aa,2) >= 0
            indices_left(point_grided(aa,3),point_grided(aa,1))=1;
%         elseif point(aa,2) <= pos_y
        elseif point(aa,2) <= 0
            indices_right(point_grided(aa,3),point_grided(aa,1))=1;
        end
    end
    
    I_front = flip(flip(indices_front,1),2);
    I_back = flip(flip(indices_back,1),2);
    I_left = flip(indices_left,1);
    I_right = flip(indices_right,1);
    
%     I_front_rgb = single(cat(3,cat(3,I_front,I_front),I_front));
%     I_back_rgb = single(cat(3,cat(3,I_back,I_back),I_back));
%     I_left_rgb = single(cat(3,cat(3,I_left,I_left),I_left));
%     I_right_rgb = single(cat(3,cat(3,I_right,I_right),I_right));
    
    image_temp_front = single(cat(3,cat(3,I_front,I_front),I_front));
    image_temp_back = single(cat(3,cat(3,I_back,I_back),I_back));
    image_temp_left = single(cat(3,cat(3,I_left,I_left),I_left));
    image_temp_right = single(cat(3,cat(3,I_right,I_right),I_right));
    
% end

    I_front_rgb = image_temp_front;
    I_back_rgb = image_temp_back;
    I_left_rgb = image_temp_left;
    I_right_rgb = image_temp_right;
    point_filtered=point_cloud;

== matlab function waypoint_generation_ptCloud_200726_mapdata_filtering_4m_2/Motor_Dynamics/Thrust &  Moment Generation  ==
  data: w_des_nomal input; force output; moment output
function [force,moment]  = fcn(w_des_nomal)

%quadrotor spec
k_f = 6.41*10^-6;
k_tau = 1.69*10^-2;
L = 0.22/2;

% 고장 시나리오 : 10초 후 모터 고장 상황 발생 시나리오   

f= zeros(4,1);
for i = 1:length(f)
    f(i) = w_des_nomal(i)^2 * k_f;
end


% Foce_total & Moment

force = [0;0;sum(f)];

roll  =  L * (f(2) - f(4));
pitch =  L * (f(3) - f(1));
yaw   =  0;
for i = 1:4
    yaw = yaw + (-1)^(i+1)*k_tau * f(i);
end

moment = [roll;pitch;yaw];

== matlab function waypoint_generation_ptCloud_200726_mapdata_filtering_4m_2/3D A* Algorithm/MATLAB Function1 ==
  data: Image input; Image_resized output; detector_image_size input
function Image_resized = fcn(Image,detector_image_size)
Image_resized = imresize(Image,[400 400]);
